simulink library "ddm"  (R2021b)
settings: Solver=VariableStepAuto  StartTime=0.0  StopTime=10.0  RelTol=1e-3
undefined symbols (not defined in the file): ADDM_FrTMTqDev_X_Nm, ADDM_RrTMTqDev_X_Nm, ENUM_ADASACCSTA_ERROR, ENUM_ADASACCSTA_OFF, ENUM_ADASACCSTA_STANDBY, ENUM_ALLOWMOV_ALLOWREADY, ENUM_APS, ENUM_BRKSTA_ERROR, ENUM_BRKSTA_OFF, ENUM_BRKSTA_ON, ENUM_BRKSW_INVALID, ENUM_BRKSW_OFF, ENUM_BRKSW_ON, ENUM_CHGPREACTERRSTA_OBCPRE, ENUM_DCDCFAULTSTA_ANYFAULTLV1, ENUM_DCDCFAULTSTA_ANYFAULTLV2, ENUM_DRIVETRAIN_AWD, ENUM_DRIVETRAIN_FWD, ENUM_DRIVETRAIN_RWD, ENUM_EDUDRTSTA_NORMAL, ENUM_EPBERROR_FAILED, ENUM_EPBSTA_APPLIED, ENUM_EPBSTA_RELEASED, ENUM_ESCAPSSta_APSUNAVAILABLE, ENUM_GEARACTUALPOSN_INVALID, ENUM_GEARACTUALPOSN_P, ENUM_HVBATTREADYPRE_READY, ENUM_HWRESETSTA_HWRESETING, ENUM_MCUWARN_LV0, ENUM_MCUWARN_LV1, ENUM_MCUWARN_LV2, ENUM_MCUWARN_LV3, ENUM_MCUWARN_NOERROR, ENUM_OBCFAULTSTA_ANYFAULT, ENUM_PAS_R2F2, ENUM_PDFAULT_BATTPDFAIL, ENUM_PDFAULT_DCDCDISABLE, ENUM_PDFAULT_MCUDISABLE, ENUM_PDFAULT_MCUDISCHRG, ENUM_POWERSTA_OFF, ENUM_POWERSTA_ON, ENUM_POWERSTA_READY, ENUM_POWERSTA_STANDBY, ENUM_PRESSINDI_LOW, ENUM_PUFAULT_BATTUPFAIL, ENUM_PUFAULT_DCDCENABLEFAIL, ENUM_PUFAULT_PRECHRGCHKFAIL, ENUM_PUFAULT_SAFETYCHKFAIL, ENUM_PWRSTASW_OFF, ENUM_PWRSTASW_OFFA, ENUM_PWRSTASW_OFFCHVCHRG, ENUM_PWRSTASW_OFFCLVCHRG, ENUM_PWRSTASW_ON, ENUM_PWRSTASW_ONHVCHRG, ENUM_PWRSTASW_READY, ENUM_PWRSTASW_STANDBY, ENUM_RAPSErrWarnSta_NORMAL, ENUM_RAPSErrWarnSta_RAPSERRLV1, ENUM_SHIFTCOMMAND_P, ENUM_SHIFTERERRSTA_PBUTTONFAILURE ... (+471)
libraries: hcu_lib x540, simulink x3
(part 19 of 26)

== system ddm/DDM/DDM/PMM/Comm err/VCU lost communication with CCU2 ==
  note: Test Detection Criteria
  note: Test Pass Criteria
  note: Diagnostics and Fault Handling
  note: Release Condition After Decision
  task_time_s : Inport
  VPMM_PowerSta_enum : Inport  Port=2
  VPMM_PwrStaSW_enum : Inport  Port=3
  VDDM_C3CCU2LCChk_flg : Inport  Port=4
  No_CAN3_BUS_OFF : Inport  Port=5
  DTC_clear_request : Inport  Port=6
  VPMM_HWResetSta_enum : Inport  Port=7
  Constant1 : Constant  Value=TRUE
  Constant10 : Constant  Value=ENUM_POWERSTA_STANDBY
  Constant11 : Constant  Value=ZERO_INT
  Constant12 : Constant  Value=KDDM_C3CCU2LCPassTO_s
  Constant13 : Constant  Value=FALSE
  Constant14 : Constant  Value=KDDM_C3CCU2LCDTC_cnt
  Constant17 : Constant  Value=KDDM_C3CCU2LCDetTO_s
  Constant2 : Constant  Value=ENUM_HWRESETSTA_HWRESETING
  Constant29 : Constant  Value=FALSE
  Constant3 : Constant  Value=ENUM_HWRESETSTA_HWRESETING
  Constant30 : Constant  Value=KDDM_CommErrDiagnosisOffSW_flg
  Constant31 : Constant  Value=ENUM_POWERSTA_OFF
  Constant32 : Constant  Value=KDDM_C3CCU2LCDTC_cnt
  Constant4 : Constant  Value=ENUM_PWRSTASW_OFF
  Constant8 : Constant  Value=KDDM_C3CCU2LCPassTO_s
  Constant9 : Constant  Value=ENUM_PWRSTASW_OFF
  DTC_Couter1 : hcu_lib/Basic_Blocks/DTC_Couter
  DTC_Info : hcu_lib/Basic_Blocks/DTC_Info
  Equal{1..4} (4 alike) : RelationalOperator  Operator=~=  OutDataTypeStr=boolean  RndMeth=Simplest
  Equal6 : RelationalOperator  OutDataTypeStr=boolean  RndMeth=Simplest
  Equal7 : RelationalOperator  Operator===  OutDataTypeStr=boolean  RndMeth=Simplest
  Equal8 : RelationalOperator  Operator===  OutDataTypeStr=boolean  RndMeth=Simplest
  Logical Operator1 : Logic  Inputs=3  AllPortsSameDT=off  OutDataTypeStr=boolean
  Logical Operator14 : Logic  Operator=OR  Inputs=4  AllPortsSameDT=off  OutDataTypeStr=boolean
  Logical Operator16 : Logic  AllPortsSameDT=off  OutDataTypeStr=boolean
  Logical Operator20 : Logic  Operator=NOT  AllPortsSameDT=off  OutDataTypeStr=boolean
  Logical Operator7 : Logic  Inputs=3  AllPortsSameDT=off  OutDataTypeStr=boolean
  Relational Operator1 : RelationalOperator  Operator=>  OutDataTypeStr=boolean  RndMeth=Simplest
  Switch1 : Switch  Criteria=u2 ~= 0
  Switch2 : Switch  Criteria=u2 ~= 0
  Switch9 : Switch  Criteria=u2 ~= 0
  Terminator : Terminator
  Test Detection Criteria1 : hcu_lib/Basic_Blocks/Test Detection Criteria
  Timer2 : hcu_lib/Basic_Blocks/Timer
  Unit Delay1 : UnitDelay  SampleTime=-1  HasFrameUpgradeWarning=on
  VDDM_C3CCU2LCDTC_raw32 : Outport
  VDDM_C3CCU2LCCFS_flg : Outport  Port=2
  wires:
  VPMM_HWResetSta_enum/1 -> [VPMM_HWResetSta_enum]
  Constant1/1 -> Switch1/3
  [VDDM_C3CCU2LCChk_flg] -> Switch1/1
  Equal3/1 -> Logical Operator1/2
  Constant3/1 -> Equal4/2
  [VPMM_HWResetSta_enum] -> Equal4/1
  [No_CAN3_BUS_OFF] -> Logical Operator1/1
  Logical Operator1/1 -> Switch1/2
  [VPMM_PwrStaSW_enum] -> Equal3/1
  Equal4/1 -> Logical Operator1/3
  Constant4/1 -> Equal3/2
  [VDDM_C3CCU2LCChk_flg] -> Switch2/1
  Equal2/1 -> Logical Operator7/3
  Constant2/1 -> Equal2/2
  Logical Operator7/1 -> Switch2/2
  Constant9/1 -> Equal1/2
  [No_CAN3_BUS_OFF] -> Logical Operator7/1
  [VPMM_PwrStaSW_enum] -> Equal1/1
  [VPMM_HWResetSta_enum] -> Equal2/1
  Constant13/1 -> Switch2/3
  Equal1/1 -> Logical Operator7/2
  [DTC_clear_request] -> DTC_Info/4
  [VDDM_C3CCU2LCDet_flg] -> DTC_Info/1
  [VDDM_C3CCU2LCCFS_flg] -> VDDM_C3CCU2LCCFS_flg/1, DTC_Info/3
  [VDDM_C3CCU2LCPass_flg] -> DTC_Info/2
  DTC_Info/1 -> VDDM_C3CCU2LCDTC_raw32/1  "VDDM_C3CCU2LCDTC_raw32"
  DTC_clear_request/1 -> [DTC_clear_request]
  No_CAN3_BUS_OFF/1 -> [No_CAN3_BUS_OFF]
  VPMM_PowerSta_enum/1 -> [VPMM_PowerSta_enum]
  VPMM_PwrStaSW_enum/1 -> [VPMM_PwrStaSW_enum]
  VDDM_C3CCU2LCChk_flg/1 -> [VDDM_C3CCU2LCChk_flg]
  task_time_s/1 -> [task_time_s]
  Constant14/1 -> Test Detection Criteria1/3
  Constant17/1 -> Test Detection Criteria1/4
  Constant8/1 -> Timer2/4
  Logical Operator16/1 -> Logical Operator14/1
  Constant10/1 -> Equal8/2
  Relational Operator1/1 -> Terminator/1  "VDDM_C3CCU2LCDFS_flg"
  [VDDM_C3CCU2LCDet_flg] -> DTC_Couter1/1
  [task_time_s] -> Test Detection Criteria1/2
  Logical Operator20/1 -> Timer2/1
  Equal7/1 -> Logical Operator16/1
  Switch1/1 -> Timer2/2, Logical Operator20/1
  [VPMM_PowerSta_enum] -> Unit Delay1/1
  Timer2/1 -> Equal6/1
  Constant12/1 -> Equal6/2
  Constant31/1 -> Equal7/2
  [DTC_clear_request] -> Logical Operator14/2
  Unit Delay1/1 -> Equal7/1
  DTC_Couter1/2 -> Relational Operator1/1  "VDDM_C3CCU2LCDTC_cnt"
  Constant11/1 -> Relational Operator1/2
  Test Detection Criteria1/1 -> [VDDM_C3CCU2LCDet_flg]  "VDDM_C3CCU2LCDet_flg"
  [VDDM_C3CCU2LCPass_flg] -> Logical Operator14/3
  Equal8/1 -> Logical Operator16/2
  Switch9/1 -> Test Detection Criteria1/1
  [VDDM_C3CCU2LCCFSRls_flg] -> DTC_Couter1/2
  Equal6/1 -> [VDDM_C3CCU2LCPass_flg]  "VDDM_C3CCU2LCPass_flg"
  Constant30/1 -> Logical Operator14/4
  Constant32/1 -> DTC_Couter1/3
  [VPMM_PowerSta_enum] -> Equal8/1
  DTC_Couter1/1 -> [VDDM_C3CCU2LCCFS_flg]  "VDDM_C3CCU2LCCFS_flg"
  [task_time_s] -> Timer2/3
  Logical Operator14/1 -> [VDDM_C3CCU2LCCFSRls_flg]  "VDDM_C3CCU2LCCFSRls_flg"
  Switch2/1 -> Switch9/3
  Constant29/1 -> Switch9/1
  [VDDM_C3CCU2LCCFSRls_flg] -> Switch9/2

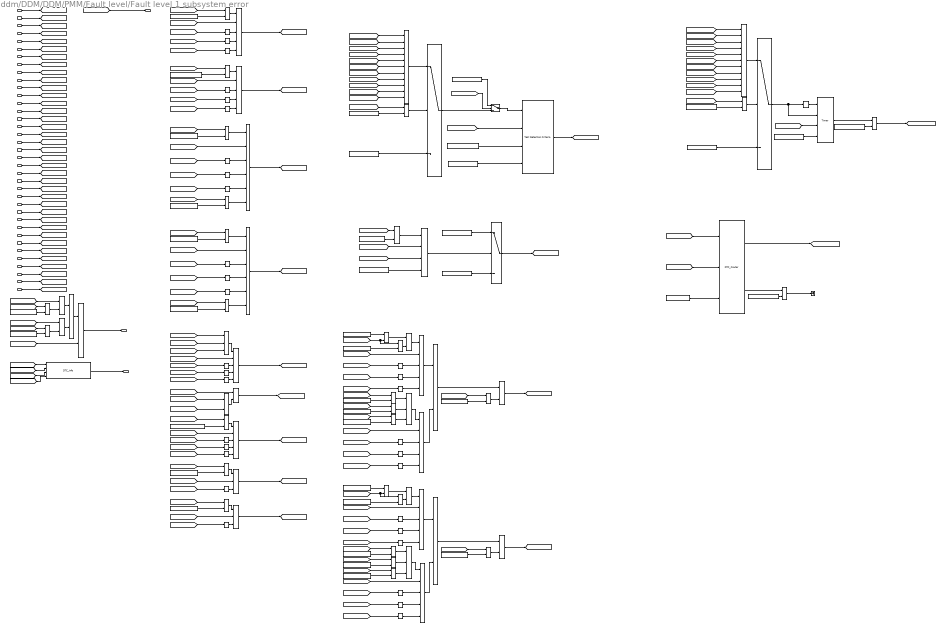
== system ddm/DDM/DDM/PMM/Fault level/Fault level 1 subsystem error ==
  note: AWD MCU Error
  note: Test Pass Criteria
  note: Test Detection Criteria
  note: Diagnostics and Fault Handling
  note: Release Condition After Failure Decision
  task_time_s : Inport
  VPMM_PowerSta_enum : Inport  Port=2
  VPMM_PwrStaSW_enum : Inport  Port=3
  VDDM_C3BMS6LCCFS_flg : Inport  Port=4
  VDDM_C3CCU2LCCFS_flg : Inport  Port=5
  VDDM_MCUF1NoComCFS_flg : Inport  Port=6
  VDDM_MCUR1NoComCFS_flg : Inport  Port=7
  VINP_BMSWarn1_flg : Inport  Port=8
  VINP_BMSWarn2_flg : Inport  Port=9
  VINP_BMSWarn3_flg : Inport  Port=10
  VINP_DCDCFaultSta_enum : Inport  Port=11
  VDDM_MCUWarnF_enum : Inport  Port=12
  VDDM_MCUWarnR_enum : Inport  Port=13
  VINP_OBCFaultSta_enum : Inport  Port=14
  VPMM_DrivetrainSelect_enum : Inport  Port=15
  DTC_clear_request : Inport  Port=16
  No_CAN3_BUS_OFF : Inport  Port=17
  VDDM_C3CCU2RCCFS_flg : Inport  Port=18
  VDDM_C3CCU2CSCFS_flg : Inport  Port=19
  VDDM_MCUR1RCErrCFS_flg : Inport  Port=20
  VDDM_MCUR1CSErrCFS_flg : Inport  Port=21
  VDDM_MCUF1RCErrCFS_flg : Inport  Port=22
  VDDM_MCUF1CSErrCFS_flg : Inport  Port=23
  VDDM_C3BMS6RCCFS_flg : Inport  Port=24
  VDDM_C3BMS6CSCFS_flg : Inport  Port=25
  No_CAN1_BUS_OFF : Inport  Port=26
  VDDM_ESC1SigErr_flg : Inport  Port=27
  VDDM_ESC5SigErr_flg : Inport  Port=28
  VINP_ShifterFailsta_enum : Inport  Port=29
  VDDM_Shifter1NoComCFS_flg : Inport  Port=30
  VDDM_Shifter1RCErrCFS_flg : Inport  Port=31
  VDDM_Shifter1CSErrCFS_flg : Inport  Port=32
  VINP_ZoneDrMalfunLevel_enum : Inport  Port=33
  No_CAN4_BUS_OFF : Inport  Port=34
  VDDM_DrVCUNoComCFS_flg : Inport  Port=35
  ZoneFrMalfunLevel_enum : Inport  Port=36
  VDDM_FrVCUNoComCFS_flg : Inport  Port=37
  AND{,1..2,4} (4 alike) : Logic  Inputs=5  AllPortsSameDT=off  OutDataTypeStr=boolean
  AND3 : Logic  AllPortsSameDT=off  OutDataTypeStr=boolean
  AND5 : Logic  Inputs=3  AllPortsSameDT=off  OutDataTypeStr=boolean
  AND6 : Logic  Inputs=3  AllPortsSameDT=off  OutDataTypeStr=boolean
  Constant : Constant  Value=KDDM_Lv1ErrDetTO_s
  Constant1 : Constant  Value=KDDM_Lv1ErrPassTO_s
  Constant{9..10,16,19,23,29} (6 alike) : Constant  Value=ENUM_MCUWARN_LV0
  Constant11 : Constant  Value=ENUM_DRIVETRAIN_AWD
  Constant12 : Constant  Value=KDDM_Lv1ErrDTC_cnt
  Constant13 : Constant  Value=ENUM_DRIVETRAIN_AWD
  Constant14 : Constant  Value=ENUM_DRIVETRAIN_FWD
  Constant15 : Constant  Value=ENUM_PWRSTASW_OFF
  Constant17 : Constant  Value=ENUM_MCUWARN_NOERROR
  Constant18 : Constant  Value=KDDM_Lv1ErrPassTO_s
  Constant2 : Constant  Value=ZERO_INT
  Constant20 : Constant  Value=ENUM_MCUWARN_LV1
  Constant{21,31..33} (4 alike) : Constant  Value=ENUM_MCUWARN_LV2
  Constant22 : Constant  Value=FALSE
  Constant24 : Constant  Value=TRUE
  Constant25 : Constant  Value=FALSE
  Constant26 : Constant  Value=ENUM_PWRSTASW_OFF
  Constant27 : Constant  Value=FALSE
  Constant28 : Constant  Value=ENUM_MCUWARN_NOERROR
  Constant3 : Constant  Value=KDDM_FaultLvDiagnosisOffSW_flg
  Constant30 : Constant  Value=ENUM_MCUWARN_LV1
  Constant36 : Constant  Value=ENUM_DCDCFAULTSTA_ANYFAULTLV1
  Constant37 : Constant  Value=ENUM_OBCFAULTSTA_ANYFAULT
  Constant39 : Constant  Value=TRUE
  Constant4 : Constant  Value=ENUM_POWERSTA_OFF
  Constant40 : Constant  Value=KDDM_Lv1ErrDTC_cnt
  Constant5 : Constant  Value=ENUM_SHIFTERERRSTA_PBUTTONFAILURE
  Constant6 : Constant  Value=ENUM_ZONEMALFUNLV_1ST
  Constant7 : Constant  Value=ENUM_ZONEMALFUNLV_1ST
  Constant8 : Constant  Value=ENUM_DRIVETRAIN_RWD
  DTC_Couter : hcu_lib/Basic_Blocks/DTC_Couter
  DTC_Info : hcu_lib/Basic_Blocks/DTC_Info
  Equal : RelationalOperator  Operator=~=  OutDataTypeStr=boolean  RndMeth=Simplest
  Equal{1,4..25} (23 alike) : RelationalOperator  Operator===  OutDataTypeStr=boolean  RndMeth=Simplest
  Equal2 : RelationalOperator  Operator=~=  OutDataTypeStr=boolean  RndMeth=Simplest
  Equal3 : RelationalOperator  OutDataTypeStr=boolean  RndMeth=Simplest
  Logical Operator{,5,10,12} (4 alike) : Logic  Inputs=5  AllPortsSameDT=off  OutDataTypeStr=boolean
  Logical Operator1 : Logic  Inputs=6  AllPortsSameDT=off  OutDataTypeStr=boolean
  Logical Operator11 : Logic  Operator=OR  AllPortsSameDT=off  OutDataTypeStr=boolean
  Logical Operator13 : Logic  Operator=OR  Inputs=3  AllPortsSameDT=off  OutDataTypeStr=boolean
  Logical Operator{2..3,9,14,17..19} (7 alike) : Logic  AllPortsSameDT=off  OutDataTypeStr=boolean
  Logical Operator15 : Logic  Operator=OR  AllPortsSameDT=off  OutDataTypeStr=boolean
  Logical Operator16 : Logic  Inputs=6  AllPortsSameDT=off  OutDataTypeStr=boolean
  Logical Operator4 : Logic  Operator=OR  AllPortsSameDT=off  OutDataTypeStr=boolean
  Logical Operator6 : Logic  Operator=NOT  AllPortsSameDT=off  OutDataTypeStr=boolean
  Logical Operator7 : Logic  Operator=OR  Inputs=3  AllPortsSameDT=off  OutDataTypeStr=boolean
  Logical Operator8 : Logic  Operator=OR  Inputs=4  AllPortsSameDT=off  OutDataTypeStr=boolean
  NOT{1..32} (32 alike) : Logic  Operator=NOT  AllPortsSameDT=off  OutDataTypeStr=boolean
  OR : Logic  Operator=OR  Inputs=3  AllPortsSameDT=off  OutDataTypeStr=boolean
  OR1 : Logic  Operator=OR  AllPortsSameDT=off  OutDataTypeStr=boolean
  OR2 : Logic  Operator=OR  Inputs=11  AllPortsSameDT=off  OutDataTypeStr=boolean
  OR3 : Logic  Operator=OR  Inputs=11  AllPortsSameDT=off  OutDataTypeStr=boolean
  Relational Operator : RelationalOperator  Operator=>  OutDataTypeStr=boolean  RndMeth=Simplest
  Relational Operator1 : RelationalOperator  OutDataTypeStr=boolean  RndMeth=Simplest
  Switch{1,4..5,9} (4 alike) : Switch  Criteria=u2 ~= 0
  Terminator : Terminator
  Test Detection Criteria : hcu_lib/Basic_Blocks/Test Detection Criteria
  Timer1 : hcu_lib/Basic_Blocks/Timer
  VDDM_Lv1ErrCFS_flg : Outport
  VDDM_Lv1ErrDTC_raw32 : Outport  Port=2
  VDDM_EDriveSysErrFaultLv1_flg : Outport  Port=3
  wires:
  task_time_s/1 -> [task_time_s]
  VPMM_PwrStaSW_enum/1 -> [VPMM_PwrStaSW_enum]
  VPMM_PowerSta_enum/1 -> [VPMM_PowerSta_enum]
  VDDM_C3CCU2LCCFS_flg/1 -> [VDDM_C3CCU2LCCFS_flg]
  VPMM_DrivetrainSelect_enum/1 -> [VPMM_DrivetrainSelect_enum]
  VDDM_MCUWarnR_enum/1 -> [VDDM_MCUWarnR_enum]
  VDDM_MCUR1NoComCFS_flg/1 -> [VDDM_MCUR1NoComCFS_flg]
  VDDM_MCUF1NoComCFS_flg/1 -> [VDDM_MCUF1NoComCFS_flg]
  VINP_BMSWarn1_flg/1 -> [VINP_BMSWarn1_flg]
  VINP_BMSWarn2_flg/1 -> [VINP_BMSWarn2_flg]
  VINP_BMSWarn3_flg/1 -> [VINP_BMSWarn3_flg]
  VINP_DCDCFaultSta_enum/1 -> [VINP_DCDCFaultSta_enum]
  VDDM_MCUWarnF_enum/1 -> [VDDM_MCUWarnF_enum]
  VINP_OBCFaultSta_enum/1 -> [VINP_OBCFaultSta_enum]
  VDDM_C3BMS6LCCFS_flg/1 -> [VDDM_C3BMS6LCCFS_flg]
  Equal4/1 -> Logical Operator8/1
  Constant1/1 -> Timer1/4
  DTC_Couter/2 -> Relational Operator/1  "VDDM_Lv1ErrDTC_cnt"
  [DTC_clear_request] -> Logical Operator8/2
  Equal3/1 -> [VDDM_Lv1ErrPass_flg]  "VDDM_Lv1ErrPass_flg"
  Timer1/1 -> Equal3/1
  Constant25/1 -> Switch4/3
  Relational Operator/1 -> Terminator/1  "VDDM_Lv1ErrDFS_flg"
  Constant12/1 -> DTC_Couter/3
  Logical Operator8/1 -> Switch4/2
  [VDDM_Lv1ErrCFSRls_flg] -> DTC_Couter/2
  Constant26/1 -> Equal/2
  Test Detection Criteria/1 -> [VDDM_Lv1ErrDet_flg]  "VDDM_Lv1ErrDet_flg"
  Constant27/1 -> Switch5/3
  Switch4/1 -> [VDDM_Lv1ErrCFSRls_flg]  "VDDM_Lv1ErrCFSRls_flg"
  [VDDM_Lv1ErrDet_flg] -> DTC_Couter/1
  Equal/1 -> Switch5/2
  [task_time_s] -> Test Detection Criteria/2
  Constant40/1 -> Test Detection Criteria/3
  Constant24/1 -> Switch4/1
  Logical Operator6/1 -> Timer1/1
  Constant18/1 -> Equal3/2
  Constant4/1 -> Equal4/2
  [VINP_DCDCFaultSta_enum] -> Equal14/1
  Constant36/1 -> Equal14/2
  [VINP_OBCFaultSta_enum] -> Equal15/1
  Constant37/1 -> Equal15/2
  Constant39/1 -> Switch1/3
  [VPMM_PowerSta_enum] -> Equal4/1
  [VPMM_PwrStaSW_enum] -> Equal/1
  [VDDM_MCUWarnR_enum] -> Equal6/1
  Constant10/1 -> Equal6/2
  Equal6/1 -> Logical Operator16/1
  DTC_clear_request/1 -> [DTC_clear_request]
  No_CAN3_BUS_OFF/1 -> [No_CAN3_BUS_OFF]
  [task_time_s] -> Timer1/3
  Constant/1 -> Test Detection Criteria/4
  Switch5/1 -> Switch9/3
  DTC_Couter/1 -> [VDDM_Lv1ErrCFS_flg]  "VDDM_Lv1ErrCFS_flg"
  Constant2/1 -> Relational Operator/2
  [VDDM_Lv1ErrPass_flg] -> Logical Operator8/3
  Constant3/1 -> Logical Operator8/4
  [VDDM_Lv1ErrCFS_flg] -> VDDM_Lv1ErrCFS_flg/1
  Equal15/1 -> AND/1
  [VDDM_C3CCU2CSCFS_flg] -> NOT3/1
  [VDDM_C3CCU2RCCFS_flg] -> NOT2/1
  [VDDM_C3CCU2LCCFS_flg] -> NOT1/1
  [No_CAN3_BUS_OFF] -> AND/2
  NOT1/1 -> AND/3
  NOT2/1 -> AND/4
  NOT3/1 -> AND/5
  AND/1 -> [VDDM_OBCFaultLv1_flg]  "VDDM_OBCFaultLv1_flg"
  [VDDM_C3CCU2CSCFS_flg] -> NOT7/1
  NOT5/1 -> AND1/3
  [VDDM_C3CCU2LCCFS_flg] -> NOT5/1
  NOT6/1 -> AND1/4
  [VDDM_C3CCU2RCCFS_flg] -> NOT6/1
  NOT7/1 -> AND1/5
  [No_CAN3_BUS_OFF] -> AND1/2
  Equal14/1 -> AND1/1
  AND1/1 -> [VDDM_DCDCFaultLv1_flg]  "VDDM_DCDCFaultLv1_flg"
  Equal5/1 -> Logical Operator16/6
  NOT11/1 -> Logical Operator16/5
  [No_CAN3_BUS_OFF] -> Logical Operator16/2
  [VDDM_MCUR1NoComCFS_flg] -> NOT9/1
  NOT9/1 -> Logical Operator16/3
  NOT10/1 -> Logical Operator16/4
  [VDDM_MCUR1CSErrCFS_flg] -> NOT11/1
  [VDDM_MCUR1RCErrCFS_flg] -> NOT10/1
  Logical Operator16/1 -> [VDDM_MCUR1FaultLv1_flg]  "VDDM_MCUR1FaultLv1_flg"
  Logical Operator1/1 -> [VDDM_MCUF1FaultLv1_flg]  "VDDM_MCUF1FaultLv1_flg"
  [VDDM_MCUF1RCErrCFS_flg] -> NOT12/1
  [VDDM_MCUF1CSErrCFS_flg] -> NOT13/1
  NOT12/1 -> Logical Operator1/4
  NOT15/1 -> Logical Operator1/3
  [VDDM_MCUF1NoComCFS_flg] -> NOT15/1
  [No_CAN3_BUS_OFF] -> Logical Operator1/2
  NOT13/1 -> Logical Operator1/5
  Equal10/1 -> Logical Operator1/6
  Equal11/1 -> Logical Operator1/1
  Constant9/1 -> Equal11/2
  [VDDM_MCUWarnF_enum] -> Equal11/1
  [VINP_BMSWarn2_flg] -> OR/2
  [VINP_BMSWarn3_flg] -> OR/3
  [VINP_BMSWarn1_flg] -> OR/1
  OR/1 -> AND2/1
  NOT18/1 -> AND2/4
  NOT19/1 -> AND2/5
  NOT17/1 -> AND2/3
  [No_CAN3_BUS_OFF] -> AND2/2
  [VDDM_C3BMS6LCCFS_flg] -> NOT17/1
  [VDDM_C3BMS6RCCFS_flg] -> NOT18/1
  [VDDM_C3BMS6CSCFS_flg] -> NOT19/1
  AND2/1 -> [VDDM_BMSFaultLv1_flg]  "VDDM_BMSFaultLv1_flg"
  [VDDM_ESC1SigErr_flg] -> OR1/1
  [VDDM_ESC5SigErr_flg] -> OR1/2
  [No_CAN1_BUS_OFF] -> AND3/1
  OR1/1 -> AND3/2
  AND3/1 -> [VDDM_ESCFaultLv1_flg]  "VDDM_ESCFaultLv1_flg"
  [VINP_ShifterFailsta_enum] -> Relational Operator1/1
  Constant5/1 -> Relational Operator1/2
  Relational Operator1/1 -> AND4/1
  NOT24/1 -> AND4/5
  NOT23/1 -> AND4/4
  NOT22/1 -> AND4/3
  [No_CAN3_BUS_OFF] -> AND4/2
  [VDDM_Shifter1NoComCFS_flg] -> NOT22/1
  [VDDM_Shifter1RCErrCFS_flg] -> NOT23/1
  [VDDM_Shifter1CSErrCFS_flg] -> NOT24/1
  AND4/1 -> [VDDM_ShifterFaultLv1_flg]  "VDDM_ShifterFaultLv1_flg"
  [VINP_ZoneDrMalfunLevel_enum] -> Equal1/1
  Constant6/1 -> Equal1/2
  Equal1/1 -> AND5/1
  [No_CAN4_BUS_OFF] -> AND5/2
  [VDDM_DrVCUNoComCFS_flg] -> NOT26/1
  NOT26/1 -> AND5/3
  AND5/1 -> [VDDM_ZoneDrFaultLv1_flg]  "VDDM_ZoneDrFaultLv1_flg"
  AND6/1 -> [VDDM_ZoneFrFaultLv1_flg]  "VDDM_ZoneFrFaultLv1_flg"
  NOT28/1 -> AND6/3
  [VDDM_FrVCUNoComCFS_flg] -> NOT28/1
  [No_CAN4_BUS_OFF] -> AND6/2
  Equal8/1 -> AND6/1
  Constant7/1 -> Equal8/2
  [ZoneFrMalfunLevel_enum] -> Equal8/1
  OR2/1 -> Switch5/1
  [VDDM_OBCFaultLv1_flg] -> OR2/1
  [VDDM_DCDCFaultLv1_flg] -> OR2/2
  [VDDM_MCUR1FaultLv1_flg] -> OR2/3
  [VDDM_MCUF1FaultLv1_flg] -> OR2/4
  [VDDM_BMSFaultLv1_flg] -> OR2/5
  [VDDM_ESCFaultLv1_flg] -> OR2/6
  [VDDM_ShifterFaultLv1_flg] -> OR2/7
  [VDDM_ZoneDrFaultLv1_flg] -> OR2/8
  [VDDM_ZoneFrFaultLv1_flg] -> OR2/9
  Equal2/1 -> Switch1/2
  [VPMM_PwrStaSW_enum] -> Equal2/1
  Constant15/1 -> Equal2/2
  Switch1/1 -> Timer1/2, Logical Operator6/1
  VDDM_C3CCU2RCCFS_flg/1 -> [VDDM_C3CCU2RCCFS_flg]
  VDDM_C3CCU2CSCFS_flg/1 -> [VDDM_C3CCU2CSCFS_flg]
  VDDM_MCUR1RCErrCFS_flg/1 -> [VDDM_MCUR1RCErrCFS_flg]
  VDDM_MCUR1CSErrCFS_flg/1 -> [VDDM_MCUR1CSErrCFS_flg]
  VDDM_MCUF1RCErrCFS_flg/1 -> [VDDM_MCUF1RCErrCFS_flg]
  VDDM_MCUF1CSErrCFS_flg/1 -> [VDDM_MCUF1CSErrCFS_flg]
  VDDM_C3BMS6RCCFS_flg/1 -> [VDDM_C3BMS6RCCFS_flg]
  VDDM_C3BMS6CSCFS_flg/1 -> [VDDM_C3BMS6CSCFS_flg]
  No_CAN1_BUS_OFF/1 -> [No_CAN1_BUS_OFF]
  VDDM_ESC1SigErr_flg/1 -> [VDDM_ESC1SigErr_flg]
  VDDM_ESC5SigErr_flg/1 -> [VDDM_ESC5SigErr_flg]
  VINP_ShifterFailsta_enum/1 -> [VINP_ShifterFailsta_enum]
  VDDM_Shifter1NoComCFS_flg/1 -> [VDDM_Shifter1NoComCFS_flg]
  VDDM_Shifter1RCErrCFS_flg/1 -> [VDDM_Shifter1RCErrCFS_flg]
  VDDM_Shifter1CSErrCFS_flg/1 -> [VDDM_Shifter1CSErrCFS_flg]
  VINP_ZoneDrMalfunLevel_enum/1 -> [VINP_ZoneDrMalfunLevel_enum]
  No_CAN4_BUS_OFF/1 -> [No_CAN4_BUS_OFF]
  VDDM_DrVCUNoComCFS_flg/1 -> [VDDM_DrVCUNoComCFS_flg]
  ZoneFrMalfunLevel_enum/1 -> [ZoneFrMalfunLevel_enum]
  VDDM_FrVCUNoComCFS_flg/1 -> [VDDM_FrVCUNoComCFS_flg]
  [VDDM_Lv1ErrDet_flg] -> DTC_Info/1
  DTC_Info/1 -> VDDM_Lv1ErrDTC_raw32/1  "VDDM_Lv1ErrDTC_raw32"
  [DTC_clear_request] -> DTC_Info/4
  [VDDM_Lv1ErrPass_flg] -> DTC_Info/2
  [VDDM_Lv1ErrCFS_flg] -> DTC_Info/3
  [VDDM_Lv1ErrCFSRls_flg] -> Switch9/2
  Constant22/1 -> Switch9/1
  Switch9/1 -> Test Detection Criteria/1
  Logical Operator/1 -> Logical Operator3/1
  Logical Operator4/1 -> Logical Operator/1
  Equal9/1 -> Logical Operator4/1
  Constant16/1 -> Equal9/1
  [VDDM_MCUWarnF_enum] -> Equal13/1, Equal9/2
  Equal13/1 -> Logical Operator4/2
  Constant17/1 -> Equal13/2
  [VDDM_MCUF1NoComCFS_flg] -> NOT14/1
  [VDDM_MCUF1CSErrCFS_flg] -> NOT8/1
  NOT8/1 -> Logical Operator/5
  [VDDM_MCUF1RCErrCFS_flg] -> NOT4/1
  NOT14/1 -> Logical Operator/3
  NOT4/1 -> Logical Operator/4
  [No_CAN3_BUS_OFF] -> Logical Operator/2
  Logical Operator5/1 -> Logical Operator3/2
  [VDDM_MCUR1NoComCFS_flg] -> NOT21/1
  [VDDM_MCUR1CSErrCFS_flg] -> NOT20/1
  NOT20/1 -> Logical Operator5/5
  [No_CAN3_BUS_OFF] -> Logical Operator5/2
  [VDDM_MCUR1RCErrCFS_flg] -> NOT16/1
  NOT21/1 -> Logical Operator5/3
  NOT16/1 -> Logical Operator5/4
  Logical Operator7/1 -> Logical Operator5/1
  Equal16/1 -> Logical Operator7/1
  Constant20/1 -> Equal17/2
  Equal17/1 -> Logical Operator7/2
  Equal18/1 -> Logical Operator7/3
  [VDDM_MCUWarnR_enum] -> Equal18/1
  Constant21/1 -> Equal18/2
  [VDDM_MCUWarnR_enum] -> Equal16/1
  Constant19/1 -> Equal16/2
  [VDDM_MCUWarnR_enum] -> Equal17/1
  Equal20/1 -> Logical Operator11/1
  [VDDM_MCUR1CSErrCFS_flg] -> NOT29/1
  NOT29/1 -> Logical Operator10/5
  NOT25/1 -> Logical Operator10/3
  [VDDM_MCUR1NoComCFS_flg] -> NOT25/1
  [No_CAN3_BUS_OFF] -> Logical Operator10/2
  NOT27/1 -> Logical Operator10/4
  Constant23/1 -> Equal20/1
  [VDDM_MCUR1RCErrCFS_flg] -> NOT27/1
  [VDDM_MCUWarnR_enum] -> Equal19/1, Equal20/2
  Logical Operator11/1 -> Logical Operator10/1
  Equal19/1 -> Logical Operator11/2
  Constant28/1 -> Equal19/2
  Logical Operator10/1 -> Logical Operator9/1
  Logical Operator12/1 -> Logical Operator9/2
  NOT31/1 -> Logical Operator12/5
  Constant29/1 -> Equal21/2
  [VDDM_MCUWarnF_enum] -> Equal22/1
  Equal23/1 -> Logical Operator13/3
  [VDDM_MCUR1RCErrCFS_flg] -> NOT30/1
  [VDDM_MCUR1CSErrCFS_flg] -> NOT31/1
  [VDDM_MCUR1NoComCFS_flg] -> NOT32/1
  Equal21/1 -> Logical Operator13/1
  Constant30/1 -> Equal22/2
  Logical Operator13/1 -> Logical Operator12/1
  Constant31/1 -> Equal23/2
  NOT30/1 -> Logical Operator12/4
  NOT32/1 -> Logical Operator12/3
  Equal22/1 -> Logical Operator13/2
  [VDDM_MCUWarnF_enum] -> Equal23/1
  [No_CAN3_BUS_OFF] -> Logical Operator12/2
  [VDDM_MCUWarnF_enum] -> Equal21/1
  [VPMM_DrivetrainSelect_enum] -> Equal5/1
  Constant8/1 -> Equal5/2
  Constant14/1 -> Equal10/2
  [VPMM_DrivetrainSelect_enum] -> Equal10/1
  Logical Operator2/1 -> [VDDM_AWDMCURrFaultLv1_flg]  "VDDM_AWDMCURrFaultLv1_flg"
  Logical Operator3/1 -> Logical Operator2/1
  Equal7/1 -> Logical Operator2/2
  [VPMM_DrivetrainSelect_enum] -> Equal7/1
  Constant11/1 -> Equal7/2
  [VPMM_DrivetrainSelect_enum] -> Equal12/1
  Constant13/1 -> Equal12/2
  Equal12/1 -> Logical Operator14/2
  Logical Operator9/1 -> Logical Operator14/1
  Logical Operator14/1 -> [VDDM_AWDMCUFrFaultLv1_flg]  "VDDM_AWDMCUFrFaultLv1_flg"
  [VDDM_AWDMCURrFaultLv1_flg] -> OR2/10
  [VDDM_AWDMCUFrFaultLv1_flg] -> OR2/11
  [VDDM_AWDMCUFrFaultLv1_flg] -> OR3/11
  [VDDM_AWDMCURrFaultLv1_flg] -> OR3/10
  [VDDM_MCUF1FaultLv1_flg] -> OR3/4
  [VDDM_ESCFaultLv1_flg] -> OR3/6
  [VDDM_DCDCFaultLv1_flg] -> OR3/2
  [VDDM_BMSFaultLv1_flg] -> OR3/5
  [VDDM_ZoneFrFaultLv1_flg] -> OR3/9
  [VDDM_ZoneDrFaultLv1_flg] -> OR3/8
  OR3/1 -> Switch1/1
  [VDDM_OBCFaultLv1_flg] -> OR3/1
  [VDDM_ShifterFaultLv1_flg] -> OR3/7
  [VDDM_MCUR1FaultLv1_flg] -> OR3/3
  [VDDM_Lv1ErrCFS_flg] -> Logical Operator17/2
  Logical Operator17/1 -> VDDM_EDriveSysErrFaultLv1_flg/1  "VDDM_EDriveSysErrFaultLv1_flg"
  Logical Operator15/1 -> Logical Operator17/1
  [VDDM_MCUWarnR_enum] -> Equal24/1
  Constant32/1 -> Equal24/2
  Logical Operator18/1 -> Logical Operator15/1
  [VDDM_AWDMCURrFaultLv1_flg] -> Logical Operator18/1
  Equal24/1 -> Logical Operator18/2
  Logical Operator19/1 -> Logical Operator15/2
  [VDDM_MCUWarnF_enum] -> Equal25/1
  Constant33/1 -> Equal25/2
  [VDDM_AWDMCUFrFaultLv1_flg] -> Logical Operator19/1
  Equal25/1 -> Logical Operator19/2

== system ddm/DDM/DDM/PMM/Fault level/Fault level 2 subsystem error ==
  note: Test Detection Criteria
  note: Diagnostics and Fault Handling
  note: Release Condition After Failure Decision
  note: Test Pass Criteria
  note: AWD MCU Error
  task_time_s : Inport
  VPMM_PowerSta_enum : Inport  Port=2
  VPMM_PwrStaSW_enum : Inport  Port=3
  VDDM_C3BMS6LCCFS_flg : Inport  Port=4
  VDDM_C3CCU2LCCFS_flg : Inport  Port=5
  VDDM_MCUF1NoComCFS_flg : Inport  Port=6
  VDDM_MCUR1NoComCFS_flg : Inport  Port=7
  VINP_BMSWarn4_flg : Inport  Port=8
  VINP_BMSWarn5_flg : Inport  Port=9
  VINP_DCDCFaultSta_enum : Inport  Port=10
  VDDM_MCUWarnF_enum : Inport  Port=11
  VDDM_MCUWarnR_enum : Inport  Port=12
  VPMM_DrivetrainSelect_enum : Inport  Port=13
  DTC_clear_request : Inport  Port=14
  No_CAN3_BUS_OFF : Inport  Port=15
  VDDM_C3CCU2RCCFS_flg : Inport  Port=16
  VDDM_C3CCU2CSCFS_flg : Inport  Port=17
  VDDM_MCUR1RCErrCFS_flg : Inport  Port=18
  VDDM_MCUR1CSErrCFS_flg : Inport  Port=19
  VDDM_MCUF1RCErrCFS_flg : Inport  Port=20
  VDDM_MCUF1CSErrCFS_flg : Inport  Port=21
  VDDM_C3BMS6RCCFS_flg : Inport  Port=22
  VDDM_C3BMS6CSCFS_flg : Inport  Port=23
  ZoneDrMalfunLevel_enum : Inport  Port=24
  No_CAN4_BUS_OFF : Inport  Port=25
  VDDM_DrVCUNoComCFS_flg : Inport  Port=26
  ZoneFrMalfunLevel_enum : Inport  Port=27
  VDDM_FrVCUNoComCFS_flg : Inport  Port=28
  AND1 : Logic  Inputs=5  AllPortsSameDT=off  OutDataTypeStr=boolean
  AND2 : Logic  Inputs=5  AllPortsSameDT=off  OutDataTypeStr=boolean
  AND5 : Logic  Inputs=3  AllPortsSameDT=off  OutDataTypeStr=boolean
  AND6 : Logic  Inputs=3  AllPortsSameDT=off  OutDataTypeStr=boolean
  Constant1 : Constant  Value=ENUM_PWRSTASW_OFF
  Constant10 : Constant  Value=ENUM_POWERSTA_STANDBY
  Constant11 : Constant  Value=ENUM_POWERSTA_OFF
  Constant12 : Constant  Value=KDDM_FaultLvDiagnosisOffSW_flg
  Constant13 : Constant  Value=ENUM_DRIVETRAIN_AWD
  Constant14 : Constant  Value=ZERO_INT
  Constant{16,23,28,31} (4 alike) : Constant  Value=ENUM_MCUWARN_LV1
  Constant19 : Constant  Value=KDDM_Lv2ErrPassTO_s
  Constant2 : Constant  Value=TRUE
  Constant20 : Constant  Value=ENUM_DRIVETRAIN_FWD
  Constant21 : Constant  Value=ENUM_DRIVETRAIN_RWD
  Constant{9,22,29,32} (4 alike) : Constant  Value=ENUM_MCUWARN_LV2
  Constant24 : Constant  Value=TRUE
  Constant25 : Constant  Value=FALSE
  Constant26 : Constant  Value=ENUM_PWRSTASW_OFF
  Constant27 : Constant  Value=FALSE
  Constant3 : Constant  Value=KDDM_Lv2ErrDetTO_s
  Constant36 : Constant  Value=ENUM_DCDCFAULTSTA_ANYFAULTLV2
  Constant4 : Constant  Value=KDDM_Lv2ErrPassTO_s
  Constant40 : Constant  Value=KDDM_Lv2ErrDTC_cnt
  Constant5 : Constant  Value=KDDM_Lv2ErrDTC_cnt
  Constant6 : Constant  Value=ENUM_ZONEMALFUNLV_2ND
  Constant7 : Constant  Value=ENUM_ZONEMALFUNLV_2ND
  Constant8 : Constant  Value=FALSE
  DTC_Couter : hcu_lib/Basic_Blocks/DTC_Couter
  DTC_Info : hcu_lib/Basic_Blocks/DTC_Info
  Delay : Delay  DelayLength=1
  Equal : RelationalOperator  Operator=~=  OutDataTypeStr=boolean  RndMeth=Simplest
  Equal1 : RelationalOperator  Operator=~=  OutDataTypeStr=boolean  RndMeth=Simplest
  Equal{2,4..6,8,10..11,13..14,17..18,22..23,25..26,28} (16 alike) : RelationalOperator  Operator===  OutDataTypeStr=boolean  RndMeth=Simplest
  Equal3 : RelationalOperator  OutDataTypeStr=boolean  RndMeth=Simplest
  Logical Operator : Logic  Inputs=5  AllPortsSameDT=off  OutDataTypeStr=boolean
  Logical Operator1 : Logic  Inputs=6  AllPortsSameDT=off  OutDataTypeStr=boolean
  Logical Operator10 : Logic  Operator=OR  AllPortsSameDT=off  OutDataTypeStr=boolean
  Logical Operator15 : Logic  Operator=OR  AllPortsSameDT=off  OutDataTypeStr=boolean
  Logical Operator{3..5,16} (4 alike) : Logic  AllPortsSameDT=off  OutDataTypeStr=boolean
  Logical Operator17 : Logic  Inputs=5  AllPortsSameDT=off  OutDataTypeStr=boolean
  Logical Operator2 : Logic  Inputs=6  AllPortsSameDT=off  OutDataTypeStr=boolean
  Logical Operator6 : Logic  Operator=NOT  AllPortsSameDT=off  OutDataTypeStr=boolean
  Logical Operator8 : Logic  Operator=OR  Inputs=4  AllPortsSameDT=off  OutDataTypeStr=boolean
  NOT{,4..21,26,28} (21 alike) : Logic  Operator=NOT  AllPortsSameDT=off  OutDataTypeStr=boolean
  OR : Logic  Operator=OR  AllPortsSameDT=off  OutDataTypeStr=boolean
  OR1 : Logic  Operator=OR  AllPortsSameDT=off  OutDataTypeStr=boolean
  OR2 : Logic  Operator=OR  Inputs=7  AllPortsSameDT=off  OutDataTypeStr=boolean
  OR3 : Logic  Operator=OR  Inputs=7  AllPortsSameDT=off  OutDataTypeStr=boolean
  OR4 : Logic  Operator=OR  AllPortsSameDT=off  OutDataTypeStr=boolean
  Relational Operator : RelationalOperator  Operator=>  OutDataTypeStr=boolean  RndMeth=Simplest
  Switch{1,4..5,9} (4 alike) : Switch  Criteria=u2 ~= 0
  Terminator : Terminator
  Test Detection Criteria : hcu_lib/Basic_Blocks/Test Detection Criteria
  Timer1 : hcu_lib/Basic_Blocks/Timer
  Unit Delay1 : UnitDelay  SampleTime=-1  HasFrameUpgradeWarning=on
  VDDM_Lv2ErrCFS_flg : Outport
  VDDM_Lv2ErrDTC_raw32 : Outport  Port=2
  wires:
  VDDM_MCUWarnF_enum/1 -> [VDDM_MCUWarnF_enum]
  VINP_DCDCFaultSta_enum/1 -> [VINP_DCDCFaultSta_enum]
  VDDM_MCUF1NoComCFS_flg/1 -> [VDDM_MCUF1NoComCFS_flg]
  VDDM_MCUR1NoComCFS_flg/1 -> [VDDM_MCUR1NoComCFS_flg]
  VDDM_MCUWarnR_enum/1 -> [VDDM_MCUWarnR_enum]
  VPMM_DrivetrainSelect_enum/1 -> [VPMM_DrivetrainSelect_enum]
  VDDM_C3CCU2LCCFS_flg/1 -> [VDDM_C3CCU2LCCFS_flg]
  VPMM_PowerSta_enum/1 -> [VPMM_PowerSta_enum]
  VPMM_PwrStaSW_enum/1 -> [VPMM_PwrStaSW_enum]
  task_time_s/1 -> [task_time_s]
  VINP_BMSWarn5_flg/1 -> [VINP_BMSWarn5_flg]
  VINP_BMSWarn4_flg/1 -> [VINP_BMSWarn4_flg]
  VDDM_C3BMS6LCCFS_flg/1 -> [VDDM_C3BMS6LCCFS_flg]
  Constant5/1 -> DTC_Couter/3
  Equal3/1 -> [VDDM_Lv2ErrPass_flg]  "VDDM_Lv2ErrPass_flg"
  Test Detection Criteria/1 -> [VDDM_Lv2ErrDet_flg]  "VDDM_Lv2ErrDet_flg"
  [task_time_s] -> Test Detection Criteria/2
  Logical Operator6/1 -> Timer1/1
  Constant36/1 -> Equal14/2
  Constant26/1 -> Equal/2
  Constant27/1 -> Switch5/3
  Logical Operator8/1 -> Switch4/2
  Switch1/1 -> Logical Operator6/1, Timer1/2
  Constant24/1 -> Switch4/1
  [VDDM_Lv2ErrDet_flg] -> DTC_Couter/1
  Constant19/1 -> Equal3/2
  Relational Operator/1 -> Terminator/1  "VDDM_Lv2ErrDFS_flg"
  Timer1/1 -> Equal3/1
  [DTC_clear_request] -> Logical Operator8/2
  DTC_Couter/1 -> [VDDM_Lv2ErrCFS_flg]  "VDDM_Lv2ErrCFS_flg"
  DTC_Couter/2 -> Relational Operator/1  "VDDM_Lv2ErrDTC_cnt"
  Constant40/1 -> Test Detection Criteria/3
  Constant25/1 -> Switch4/3
  [VINP_DCDCFaultSta_enum] -> Equal14/1
  Switch4/1 -> [VDDM_Lv2ErrCFSRls_flg]  "VDDM_Lv2ErrCFSRls_flg"
  Constant4/1 -> Timer1/4
  [VPMM_PwrStaSW_enum] -> Equal/1
  DTC_clear_request/1 -> [DTC_clear_request]
  No_CAN3_BUS_OFF/1 -> [No_CAN3_BUS_OFF]
  [task_time_s] -> Timer1/3
  Constant3/1 -> Test Detection Criteria/4
  Switch5/1 -> Switch9/3
  Constant14/1 -> Relational Operator/2
  [VDDM_Lv2ErrCFSRls_flg] -> DTC_Couter/2
  Logical Operator3/1 -> Logical Operator8/3
  [VDDM_Lv2ErrPass_flg] -> Logical Operator3/1
  NOT/1 -> Logical Operator3/2
  Delay/1 -> NOT/1
  [VDDM_Lv2ErrCFS_flg] -> Delay/1
  Constant12/1 -> Logical Operator8/4
  Equal/1 -> Switch5/2
  NOT5/1 -> AND1/3
  [VDDM_C3CCU2LCCFS_flg] -> NOT5/1
  [VDDM_C3CCU2CSCFS_flg] -> NOT7/1
  NOT7/1 -> AND1/5
  [VDDM_C3CCU2RCCFS_flg] -> NOT6/1
  NOT6/1 -> AND1/4
  Equal14/1 -> AND1/1
  [No_CAN3_BUS_OFF] -> AND1/2
  AND1/1 -> [VDDM_DCDCFaultLv2_flg]  "VDDM_DCDCFaultLv2_flg"
  Constant22/1 -> Equal23/2
  [VDDM_MCUF1NoComCFS_flg] -> NOT15/1
  Equal25/1 -> Logical Operator2/6
  NOT11/1 -> Logical Operator2/5
  [VDDM_MCUR1NoComCFS_flg] -> NOT9/1
  Constant16/1 -> Equal26/2
  Logical Operator2/1 -> [VDDM_MCUR1FaultLv2_flg]  "VDDM_MCUR1FaultLv2_flg"
  [No_CAN3_BUS_OFF] -> Logical Operator2/2
  Logical Operator1/1 -> [VDDM_MCUF1FaultLv2_flg]  "VDDM_MCUF1FaultLv2_flg"
  [VDDM_MCUR1CSErrCFS_flg] -> NOT11/1
  [No_CAN3_BUS_OFF] -> Logical Operator1/2
  [VDDM_MCUF1RCErrCFS_flg] -> NOT12/1
  NOT13/1 -> Logical Operator1/5
  NOT12/1 -> Logical Operator1/4
  [VDDM_MCUF1CSErrCFS_flg] -> NOT13/1
  Equal22/1 -> Logical Operator1/6
  [VDDM_MCUR1RCErrCFS_flg] -> NOT10/1
  NOT10/1 -> Logical Operator2/4
  NOT15/1 -> Logical Operator1/3
  Equal26/1 -> OR4/1
  [VDDM_MCUWarnF_enum] -> Equal23/1
  NOT9/1 -> Logical Operator2/3
  [VDDM_MCUWarnR_enum] -> Equal26/1
  Constant28/1 -> Equal28/2
  Equal28/1 -> OR/1
  Equal23/1 -> OR/2
  OR/1 -> Logical Operator1/1
  NOT17/1 -> AND2/3
  AND2/1 -> [VDDM_BMSFaultLv2_flg]  "VDDM_BMSFaultLv2_flg"
  [VDDM_C3BMS6RCCFS_flg] -> NOT18/1
  OR1/1 -> AND2/1
  [No_CAN3_BUS_OFF] -> AND2/2
  NOT18/1 -> AND2/4
  [VDDM_C3BMS6LCCFS_flg] -> NOT17/1
  [VINP_BMSWarn5_flg] -> OR1/2
  [VINP_BMSWarn4_flg] -> OR1/1
  [VDDM_C3BMS6CSCFS_flg] -> NOT19/1
  NOT19/1 -> AND2/5
  [VDDM_DCDCFaultLv2_flg] -> OR2/1
  [VDDM_MCUR1FaultLv2_flg] -> OR2/2
  [VDDM_MCUF1FaultLv2_flg] -> OR2/3
  [VDDM_BMSFaultLv2_flg] -> OR2/4
  OR2/1 -> Switch5/1
  OR3/1 -> Switch1/1
  Equal1/1 -> Switch1/2
  [VPMM_PwrStaSW_enum] -> Equal1/1
  Constant2/1 -> Switch1/3
  Constant1/1 -> Equal1/2
  [VDDM_Lv2ErrCFS_flg] -> VDDM_Lv2ErrCFS_flg/1
  VDDM_C3CCU2RCCFS_flg/1 -> [VDDM_C3CCU2RCCFS_flg]
  VDDM_C3CCU2CSCFS_flg/1 -> [VDDM_C3CCU2CSCFS_flg]
  VDDM_MCUR1RCErrCFS_flg/1 -> [VDDM_MCUR1RCErrCFS_flg]
  VDDM_MCUR1CSErrCFS_flg/1 -> [VDDM_MCUR1CSErrCFS_flg]
  VDDM_MCUF1RCErrCFS_flg/1 -> [VDDM_MCUF1RCErrCFS_flg]
  VDDM_MCUF1CSErrCFS_flg/1 -> [VDDM_MCUF1CSErrCFS_flg]
  VDDM_C3BMS6RCCFS_flg/1 -> [VDDM_C3BMS6RCCFS_flg]
  VDDM_C3BMS6CSCFS_flg/1 -> [VDDM_C3BMS6CSCFS_flg]
  [No_CAN4_BUS_OFF] -> AND5/2
  [ZoneFrMalfunLevel_enum] -> Equal8/1
  Constant7/1 -> Equal8/2
  Equal8/1 -> AND6/1
  NOT26/1 -> AND5/3
  [ZoneDrMalfunLevel_enum] -> Equal2/1
  AND6/1 -> [VDDM_ZoneFrFaultLv2_flg]  "VDDM_ZoneFrFaultLv2_flg"
  [No_CAN4_BUS_OFF] -> AND6/2
  AND5/1 -> [VDDM_ZoneDrFaultLv2_flg]  "VDDM_ZoneDrFaultLv2_flg"
  [VDDM_DrVCUNoComCFS_flg] -> NOT26/1
  Constant6/1 -> Equal2/2
  Equal2/1 -> AND5/1
  [VDDM_FrVCUNoComCFS_flg] -> NOT28/1
  NOT28/1 -> AND6/3
  [VDDM_ZoneDrFaultLv2_flg] -> OR2/5
  [VDDM_ZoneFrFaultLv2_flg] -> OR2/6
  ZoneDrMalfunLevel_enum/1 -> [ZoneDrMalfunLevel_enum]
  No_CAN4_BUS_OFF/1 -> [No_CAN4_BUS_OFF]
  VDDM_DrVCUNoComCFS_flg/1 -> [VDDM_DrVCUNoComCFS_flg]
  ZoneFrMalfunLevel_enum/1 -> [ZoneFrMalfunLevel_enum]
  VDDM_FrVCUNoComCFS_flg/1 -> [VDDM_FrVCUNoComCFS_flg]
  [DTC_clear_request] -> DTC_Info/4
  [VDDM_Lv2ErrDet_flg] -> DTC_Info/1
  [VDDM_Lv2ErrPass_flg] -> DTC_Info/2
  DTC_Info/1 -> VDDM_Lv2ErrDTC_raw32/1  "VDDM_Lv2ErrDTC_raw32"
  [VDDM_Lv2ErrCFS_flg] -> DTC_Info/3
  [VDDM_Lv2ErrCFSRls_flg] -> Switch9/2
  Constant8/1 -> Switch9/1
  Switch9/1 -> Test Detection Criteria/1
  OR4/1 -> Logical Operator2/1
  Equal5/1 -> OR4/2
  [VDDM_MCUWarnR_enum] -> Equal5/1
  Constant9/1 -> Equal5/2
  [VPMM_PowerSta_enum] -> Equal6/1
  Constant10/1 -> Equal6/2
  Equal6/1 -> Logical Operator16/2
  Equal4/1 -> Logical Operator16/1
  Constant11/1 -> Equal4/2
  Unit Delay1/1 -> Equal4/1
  [VPMM_PowerSta_enum] -> Unit Delay1/1
  Logical Operator16/1 -> Logical Operator8/1
  [VDDM_MCUF1RCErrCFS_flg] -> NOT4/1
  [VDDM_MCUF1NoComCFS_flg] -> NOT14/1
  [VDDM_MCUR1RCErrCFS_flg] -> NOT16/1
  NOT21/1 -> Logical Operator17/3
  [VDDM_MCUWarnR_enum] -> Equal17/1
  Constant31/1 -> Equal17/2
  NOT20/1 -> Logical Operator17/5
  NOT16/1 -> Logical Operator17/4
  [VDDM_MCUF1CSErrCFS_flg] -> NOT8/1
  NOT4/1 -> Logical Operator/4
  [No_CAN3_BUS_OFF] -> Logical Operator17/2
  Equal18/1 -> Logical Operator10/2
  NOT8/1 -> Logical Operator/5
  NOT14/1 -> Logical Operator/3
  Logical Operator15/1 -> Logical Operator/1
  Equal13/1 -> Logical Operator15/2
  [VDDM_MCUWarnR_enum] -> Equal18/1
  [VPMM_DrivetrainSelect_enum] -> Equal10/1
  Logical Operator17/1 -> Logical Operator5/2
  [VDDM_MCUR1CSErrCFS_flg] -> NOT20/1
  [No_CAN3_BUS_OFF] -> Logical Operator/2
  [VDDM_MCUR1NoComCFS_flg] -> NOT21/1
  Constant32/1 -> Equal18/2
  Logical Operator/1 -> Logical Operator5/1
  Constant13/1 -> Equal10/2
  Equal10/1 -> Logical Operator4/2
  Constant29/1 -> Equal13/2
  Logical Operator5/1 -> Logical Operator4/1
  Logical Operator10/1 -> Logical Operator17/1
  Logical Operator4/1 -> [VDDM_AWDMCUFaultLv2_flg]  "VDDM_AWDMCUFaultLv2_flg"
  Equal11/1 -> Logical Operator15/1
  Constant23/1 -> Equal11/2
  [VDDM_MCUWarnF_enum] -> Equal11/1
  [VDDM_MCUWarnF_enum] -> Equal13/1
  Equal17/1 -> Logical Operator10/1
  Constant21/1 -> Equal25/2
  [VPMM_DrivetrainSelect_enum] -> Equal25/1
  Constant20/1 -> Equal22/2
  [VPMM_DrivetrainSelect_enum] -> Equal22/1
  [VDDM_AWDMCUFaultLv2_flg] -> OR2/7
  [VDDM_ZoneDrFaultLv2_flg] -> OR3/5
  [VDDM_MCUR1FaultLv2_flg] -> OR3/2
  [VDDM_MCUF1FaultLv2_flg] -> OR3/3
  [VDDM_BMSFaultLv2_flg] -> OR3/4
  [VDDM_DCDCFaultLv2_flg] -> OR3/1
  [VDDM_AWDMCUFaultLv2_flg] -> OR3/7
  [VDDM_ZoneFrFaultLv2_flg] -> OR3/6
  [VDDM_MCUWarnF_enum] -> Equal28/1

== system ddm/DDM/DDM/PMM/Fault level/Fault level 3 subsystem error ==
  note: Test Pass Criteria
  note: Test Detection Criteria
  note: Diagnostics and Fault Handling
  note: Release Condition After Failure Decision
  task_time_s : Inport
  VPMM_PowerSta_enum : Inport  Port=2
  VPMM_PwrStaSW_enum : Inport  Port=3
  VDDM_C3BMS6LCCFS_flg : Inport  Port=4
  VDDM_MCUF1NoComCFS_flg : Inport  Port=5
  VDDM_MCUR1NoComCFS_flg : Inport  Port=6
  VINP_BMSWarn6_flg : Inport  Port=7
  VDDM_MCUWarnF_enum : Inport  Port=8
  VDDM_MCUWarnR_enum : Inport  Port=9
  VPMM_DrivetrainSelect_enum : Inport  Port=10
  DTC_clear_request : Inport  Port=11
  No_CAN3_BUS_OFF : Inport  Port=12
  VDDM_MCUR1RCErrCFS_flg : Inport  Port=13
  VDDM_MCUR1CSErrCFS_flg : Inport  Port=14
  VDDM_MCUF1RCErrCFS_flg : Inport  Port=15
  VDDM_MCUF1CSErrCFS_flg : Inport  Port=16
  VDDM_C3BMS6RCCFS_flg : Inport  Port=17
  VDDM_C3BMS6CSCFS_flg : Inport  Port=18
  ZoneDrMalfunLevel_enum : Inport  Port=19
  No_CAN4_BUS_OFF : Inport  Port=20
  VDDM_DrVCUNoComCFS_flg : Inport  Port=21
  ZoneFrMalfunLevel_enum : Inport  Port=22
  VDDM_FrVCUNoComCFS_flg : Inport  Port=23
  AND2 : Logic  Inputs=5  AllPortsSameDT=off  OutDataTypeStr=boolean
  AND5 : Logic  Inputs=3  AllPortsSameDT=off  OutDataTypeStr=boolean
  AND6 : Logic  Inputs=3  AllPortsSameDT=off  OutDataTypeStr=boolean
  Constant1 : Constant  Value=ENUM_PWRSTASW_OFF
  Constant10 : Constant  Value=ENUM_MCUWARN_LV3
  Constant11 : Constant  Value=ENUM_DRIVETRAIN_AWD
  Constant12 : Constant  Value=KDDM_FaultLvDiagnosisOffSW_flg
  Constant13 : Constant  Value=ENUM_DRIVETRAIN_RWD
  Constant14 : Constant  Value=ZERO_INT
  Constant15 : Constant  Value=ENUM_DRIVETRAIN_AWD
  Constant16 : Constant  Value=ENUM_DRIVETRAIN_FWD
  Constant17 : Constant  Value=ENUM_MCUWARN_LV3
  Constant18 : Constant  Value=KDDM_Lv3ErrPassTO_s
  Constant2 : Constant  Value=TRUE
  Constant20 : Constant  Value=ENUM_ZONEMALFUNLV_3RD
  Constant21 : Constant  Value=ENUM_ZONEMALFUNLV_3RD
  Constant22 : Constant  Value=FALSE
  Constant24 : Constant  Value=TRUE
  Constant25 : Constant  Value=FALSE
  Constant26 : Constant  Value=ENUM_PWRSTASW_OFF
  Constant27 : Constant  Value=FALSE
  Constant3 : Constant  Value=KDDM_Lv3ErrDetTO_s
  Constant4 : Constant  Value=KDDM_Lv3ErrPassTO_s
  Constant40 : Constant  Value=KDDM_Lv3ErrDTC_cnt
  Constant5 : Constant  Value=KDDM_Lv3ErrDTC_cnt
  Constant6 : Constant  Value=ENUM_POWERSTA_STANDBY
  Constant8 : Constant  Value=ENUM_POWERSTA_OFF
  DTC_Couter : hcu_lib/Basic_Blocks/DTC_Couter
  DTC_Info : hcu_lib/Basic_Blocks/DTC_Info
  Delay : Delay  DelayLength=1
  Equal : RelationalOperator  Operator=~=  OutDataTypeStr=boolean  RndMeth=Simplest
  Equal1 : RelationalOperator  Operator=~=  OutDataTypeStr=boolean  RndMeth=Simplest
  Equal{4,6,8..9,11..13,16..18} (10 alike) : RelationalOperator  Operator===  OutDataTypeStr=boolean  RndMeth=Simplest
  Equal3 : RelationalOperator  OutDataTypeStr=boolean  RndMeth=Simplest
  Logical Operator1 : Logic  Inputs=6  AllPortsSameDT=off  OutDataTypeStr=boolean
  Logical Operator16 : Logic  AllPortsSameDT=off  OutDataTypeStr=boolean
  Logical Operator2 : Logic  Operator=OR  AllPortsSameDT=off  OutDataTypeStr=boolean
  Logical Operator21 : Logic  AllPortsSameDT=off  OutDataTypeStr=boolean
  Logical Operator3 : Logic  Inputs=6  AllPortsSameDT=off  OutDataTypeStr=boolean
  Logical Operator6 : Logic  Operator=NOT  AllPortsSameDT=off  OutDataTypeStr=boolean
  Logical Operator8 : Logic  Operator=OR  Inputs=4  AllPortsSameDT=off  OutDataTypeStr=boolean
  Logical Operator9 : Logic  Operator=OR  AllPortsSameDT=off  OutDataTypeStr=boolean
  NOT{,9..13,15,17..19,26,28} (12 alike) : Logic  Operator=NOT  AllPortsSameDT=off  OutDataTypeStr=boolean
  OR : Logic  Operator=OR  Inputs=5  AllPortsSameDT=off  OutDataTypeStr=boolean
  OR1 : Logic  Operator=OR  Inputs=5  AllPortsSameDT=off  OutDataTypeStr=boolean
  Relational Operator : RelationalOperator  Operator=>  OutDataTypeStr=boolean  RndMeth=Simplest
  Switch{1,4..5,9} (4 alike) : Switch  Criteria=u2 ~= 0
  Terminator : Terminator
  Test Detection Criteria : hcu_lib/Basic_Blocks/Test Detection Criteria
  Timer1 : hcu_lib/Basic_Blocks/Timer
  Unit Delay1 : UnitDelay  SampleTime=-1  HasFrameUpgradeWarning=on
  VDDM_Lv3ErrCFS_flg : Outport
  VDDM_Lv3ErrDTC_raw32 : Outport  Port=2
  wires:
  VINP_BMSWarn6_flg/1 -> [VINP_BMSWarn6_flg]
  task_time_s/1 -> [task_time_s]
  VPMM_PwrStaSW_enum/1 -> [VPMM_PwrStaSW_enum]
  VPMM_PowerSta_enum/1 -> [VPMM_PowerSta_enum]
  VPMM_DrivetrainSelect_enum/1 -> [VPMM_DrivetrainSelect_enum]
  VDDM_MCUWarnR_enum/1 -> [VDDM_MCUWarnR_enum]
  VDDM_MCUR1NoComCFS_flg/1 -> [VDDM_MCUR1NoComCFS_flg]
  VDDM_MCUF1NoComCFS_flg/1 -> [VDDM_MCUF1NoComCFS_flg]
  VDDM_MCUWarnF_enum/1 -> [VDDM_MCUWarnF_enum]
  VDDM_C3BMS6LCCFS_flg/1 -> [VDDM_C3BMS6LCCFS_flg]
  Constant5/1 -> DTC_Couter/3
  Equal3/1 -> [VDDM_Lv3ErrPass_flg]  "VDDM_Lv3ErrPass_flg"
  Test Detection Criteria/1 -> [VDDM_Lv3ErrDet_flg]  "VDDM_Lv3ErrDet_flg"
  [task_time_s] -> Test Detection Criteria/2
  Logical Operator6/1 -> Timer1/1
  Logical Operator8/1 -> Switch4/2
  Constant27/1 -> Switch5/3
  Switch1/1 -> Logical Operator6/1, Timer1/2
  Constant24/1 -> Switch4/1
  [VDDM_Lv3ErrDet_flg] -> DTC_Couter/1
  Equal/1 -> Switch5/2
  Constant18/1 -> Equal3/2
  Relational Operator/1 -> Terminator/1  "VDDM_Lv3ErrDFS_flg"
  Constant26/1 -> Equal/2
  Timer1/1 -> Equal3/1
  [DTC_clear_request] -> Logical Operator8/2
  DTC_Couter/1 -> [VDDM_Lv3ErrCFS_flg]  "VDDM_Lv3ErrCFS_flg"
  DTC_Couter/2 -> Relational Operator/1  "VDDM_Lv3ErrDTC_cnt"
  Constant40/1 -> Test Detection Criteria/3
  Constant25/1 -> Switch4/3
  Switch4/1 -> [VDDM_Lv3ErrCFSRls_flg]  "VDDM_Lv3ErrCFSRls_flg"
  Constant4/1 -> Timer1/4
  [VPMM_PwrStaSW_enum] -> Equal/1
  DTC_clear_request/1 -> [DTC_clear_request]
  No_CAN3_BUS_OFF/1 -> [No_CAN3_BUS_OFF]
  [task_time_s] -> Timer1/3
  Constant3/1 -> Test Detection Criteria/4
  Switch5/1 -> Switch9/3
  [VDDM_Lv3ErrPass_flg] -> Logical Operator21/1
  Constant12/1 -> Logical Operator8/4
  Delay/1 -> NOT/1
  NOT/1 -> Logical Operator21/2
  [VDDM_Lv3ErrCFS_flg] -> Delay/1
  Logical Operator21/1 -> Logical Operator8/3
  [VDDM_Lv3ErrCFSRls_flg] -> DTC_Couter/2
  Constant14/1 -> Relational Operator/2
  [VDDM_MCUR1RCErrCFS_flg] -> NOT10/1
  NOT11/1 -> Logical Operator1/5
  Logical Operator1/1 -> [VDDM_MCUR1FaultLv3_flg]  "VDDM_MCUR1FaultLv3_flg"
  Logical Operator2/1 -> Logical Operator1/6
  [VDDM_MCUR1CSErrCFS_flg] -> NOT11/1
  [No_CAN3_BUS_OFF] -> Logical Operator1/2
  NOT10/1 -> Logical Operator1/4
  [VPMM_DrivetrainSelect_enum] -> Equal18/1, Equal16/2
  [VDDM_MCUWarnR_enum] -> Equal17/1
  Constant10/1 -> Equal17/2
  Constant13/1 -> Equal16/1
  Constant11/1 -> Equal18/2
  [VDDM_MCUR1NoComCFS_flg] -> NOT9/1
  Equal16/1 -> Logical Operator2/1
  Equal18/1 -> Logical Operator2/2
  NOT9/1 -> Logical Operator1/3
  Equal17/1 -> Logical Operator1/1
  NOT15/1 -> Logical Operator3/3
  Equal12/1 -> Logical Operator3/1
  [VDDM_MCUWarnF_enum] -> Equal12/1
  [VPMM_DrivetrainSelect_enum] -> Equal13/1, Equal11/2
  [VDDM_MCUF1RCErrCFS_flg] -> NOT12/1
  Equal11/1 -> Logical Operator9/1
  Logical Operator3/1 -> [VDDM_MCUF1FaultLv3_flg]  "VDDM_MCUF1FaultLv3_flg"
  NOT12/1 -> Logical Operator3/4
  NOT13/1 -> Logical Operator3/5
  [VDDM_MCUF1NoComCFS_flg] -> NOT15/1
  Logical Operator9/1 -> Logical Operator3/6
  [No_CAN3_BUS_OFF] -> Logical Operator3/2
  Constant16/1 -> Equal11/1
  Equal13/1 -> Logical Operator9/2
  Constant17/1 -> Equal12/2
  [VDDM_MCUF1CSErrCFS_flg] -> NOT13/1
  [VDDM_C3BMS6LCCFS_flg] -> NOT17/1
  [No_CAN3_BUS_OFF] -> AND2/2
  [VDDM_C3BMS6RCCFS_flg] -> NOT18/1
  NOT28/1 -> AND6/3
  [VDDM_FrVCUNoComCFS_flg] -> NOT28/1
  AND6/1 -> [VDDM_ZoneFrFaultLv3_flg]  "VDDM_ZoneFrFaultLv3_flg"
  [No_CAN4_BUS_OFF] -> AND6/2
  Equal8/1 -> AND5/1
  Constant20/1 -> Equal8/2
  NOT17/1 -> AND2/3
  AND2/1 -> [VDDM_BMSFaultLv3_flg]  "VDDM_BMSFaultLv3_flg"
  [VDDM_DrVCUNoComCFS_flg] -> NOT26/1
  [VINP_BMSWarn6_flg] -> AND2/1
  [ZoneDrMalfunLevel_enum] -> Equal8/1
  NOT26/1 -> AND5/3
  Equal9/1 -> AND6/1
  [ZoneFrMalfunLevel_enum] -> Equal9/1
  [No_CAN4_BUS_OFF] -> AND5/2
  NOT18/1 -> AND2/4
  Constant21/1 -> Equal9/2
  NOT19/1 -> AND2/5
  [VDDM_C3BMS6CSCFS_flg] -> NOT19/1
  AND5/1 -> [VDDM_ZoneDrFaultLv3_flg]  "VDDM_ZoneDrFaultLv3_flg"
  Constant15/1 -> Equal13/2
  [VDDM_MCUR1FaultLv3_flg] -> OR/1
  [VDDM_MCUF1FaultLv3_flg] -> OR/2
  [VDDM_BMSFaultLv3_flg] -> OR/3
  [VDDM_ZoneDrFaultLv3_flg] -> OR/4
  [VDDM_ZoneFrFaultLv3_flg] -> OR/5
  OR/1 -> Switch5/1
  [VDDM_MCUR1FaultLv3_flg] -> OR1/1
  [VDDM_BMSFaultLv3_flg] -> OR1/3
  Equal1/1 -> Switch1/2
  [VDDM_MCUF1FaultLv3_flg] -> OR1/2
  [VDDM_ZoneDrFaultLv3_flg] -> OR1/4
  [VPMM_PwrStaSW_enum] -> Equal1/1
  Constant1/1 -> Equal1/2
  Constant2/1 -> Switch1/3
  [VDDM_ZoneFrFaultLv3_flg] -> OR1/5
  OR1/1 -> Switch1/1
  [VDDM_Lv3ErrCFS_flg] -> VDDM_Lv3ErrCFS_flg/1
  VDDM_MCUR1RCErrCFS_flg/1 -> [VDDM_MCUR1RCErrCFS_flg]
  VDDM_MCUR1CSErrCFS_flg/1 -> [VDDM_MCUR1CSErrCFS_flg]
  VDDM_MCUF1RCErrCFS_flg/1 -> [VDDM_MCUF1RCErrCFS_flg]
  VDDM_MCUF1CSErrCFS_flg/1 -> [VDDM_MCUF1CSErrCFS_flg]
  VDDM_C3BMS6RCCFS_flg/1 -> [VDDM_C3BMS6RCCFS_flg]
  VDDM_C3BMS6CSCFS_flg/1 -> [VDDM_C3BMS6CSCFS_flg]
  ZoneDrMalfunLevel_enum/1 -> [ZoneDrMalfunLevel_enum]
  No_CAN4_BUS_OFF/1 -> [No_CAN4_BUS_OFF]
  VDDM_DrVCUNoComCFS_flg/1 -> [VDDM_DrVCUNoComCFS_flg]
  ZoneFrMalfunLevel_enum/1 -> [ZoneFrMalfunLevel_enum]
  VDDM_FrVCUNoComCFS_flg/1 -> [VDDM_FrVCUNoComCFS_flg]
  [VDDM_Lv3ErrDet_flg] -> DTC_Info/1
  [DTC_clear_request] -> DTC_Info/4
  [VDDM_Lv3ErrPass_flg] -> DTC_Info/2
  [VDDM_Lv3ErrCFS_flg] -> DTC_Info/3
  DTC_Info/1 -> VDDM_Lv3ErrDTC_raw32/1  "VDDM_Lv3ErrDTC_raw32"
  [VDDM_Lv3ErrCFSRls_flg] -> Switch9/2
  Constant22/1 -> Switch9/1
  Switch9/1 -> Test Detection Criteria/1
  [VPMM_PowerSta_enum] -> Equal6/1
  Constant6/1 -> Equal6/2
  Equal6/1 -> Logical Operator16/2
  Equal4/1 -> Logical Operator16/1
  Constant8/1 -> Equal4/2
  Unit Delay1/1 -> Equal4/1
  [VPMM_PowerSta_enum] -> Unit Delay1/1
  Logical Operator16/1 -> Logical Operator8/1
